simulink model "FILTRE_KALMAN_Design"  (R2024a)
settings: Solver=FixedStepAuto  StartTime=0.0  StopTime=10.0  FixedStep=0.01  RelTol=1e-3
values from neighbouring files (symbols this model uses):
  A = [0 0 1 0; 0 0 0 1; 0 aa -bb -cc; 0 dd -ee -ff]    [Init_Setup.m]
  b = 0.00007892    (= 7.892e-05)    [Init_Setup.m]
  B = [0;0; mm; nn]    [Init_Setup.m]
  c = 0.63    [Init_Setup.m]
  C = eye(4)    [Init_Setup.m]
  D = [0 0 0 0]'    [Init_Setup.m]
  g = 9.81    [Init_Setup.m]
  I = 0.0007176    [Init_Setup.m]
  kb = 0.031    [Init_Setup.m]
  kt = 0.031    [Init_Setup.m]
  l = 0.2    [Init_Setup.m]
  M = 0.136    [Init_Setup.m]
  m = 0.1    [Init_Setup.m]
  r = 0.006    [Init_Setup.m]
  Rm = 12.5    [Init_Setup.m]
undefined symbols (not defined in the file or in its folder): Continuous, Time
libraries: simulink x2, ctrlSharedLib x1
settings Model: Creator=jitendra  LastModifiedBy=USER
settings SolverCC: AlgebraicLoopSolver=TrustRegion
settings DataIOCC: ExternalInput=getinputstruct(op_trim1)  InitialState=getstatestruct(op_trim1)  ReturnWorkspaceOutputs=off
settings DebuggingCC: UnconnectedInputMsg=warning  UnconnectedOutputMsg=warning  UnconnectedLineMsg=warning  ArithmeticOperatorsInVariantConditions=warning
settings ModelReferenceCC: EnableRefExpFcnMdlSchedulingChecks=on
settings SFSimCC: SimUseLocalCustomCode=off  CustomCodeUndefinedFunction=UseInterfaceOnly
settings RTWCC: RTWUseLocalCustomCode=off  GPUComputeCapability=3.5

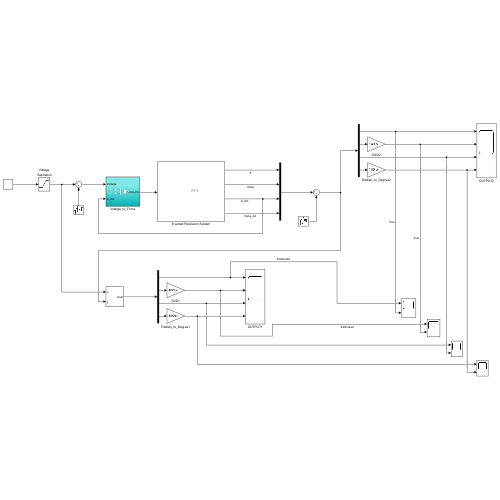
[thumbnail: Simulink's stored preview of the top-level diagram]
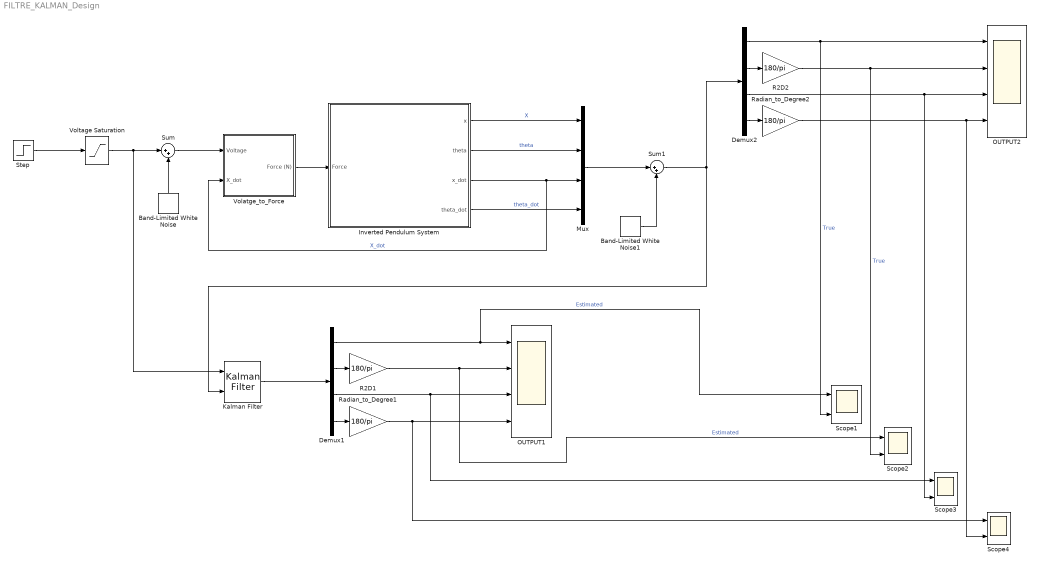
== system FILTRE_KALMAN_Design ==
  Band-Limited White Noise : simulink/Sources/Band-Limited White Noise  Cov=[0.000015]  Ts=0.1  seed=[23341]
  Band-Limited White Noise1 : simulink/Sources/Band-Limited White Noise  Cov=[0.00015]  Ts=0.1  seed=[23341]
  Demux1 : Demux
  Demux2 : Demux
  Inverted Pendulum System : Subsystem
      mask Display: image('ip_model.png');
  Kalman Filter : ctrlSharedLib/Kalman Filter  TimeDomain=Continuous-Time  UseCurrentEstimator=on  ModelSource=Individual A, B, C, D matrices  ModelSourceVariable=ss(0.95,1,1,0,1)  A=A  B=B  C=C  D=D  NumberOfStates=1  NumberOfInputs=1  NumberOfOutputs=1  InitialEstimateSource=Dialog  X0=0  P0=10  UseK=off  UseGH=off  NumberOfProcessNoiseInputs=1  G=1  TimeInvariantG=on  H=0  TimeInvariantH=on  Q=0.05  TimeInvariantQ=on  R=1  TimeInvariantR=on  N=0  TimeInvariantN=on  AddInputPort=on  AddEnablePort=off  OutputEstimatedY=off  OutputP=off  Ts=-1
  Mux : Mux
  OUTPUT1 : Scope  NumInputPorts=4
  OUTPUT2 : Scope  NumInputPorts=4
  R2D1 : Gain  Gain=180/pi
  R2D2 : Gain  Gain=180/pi
  Radian_to_Degree1 : Gain  Gain=180/pi
  Radian_to_Degree2 : Gain  Gain=180/pi
  Scope{1..4} (4 alike) : Scope  NumInputPorts=2
  Step : Step  SampleTime=0
  Sum : Sum  Inputs=|++
  Sum1 : Sum  Inputs=|++
  Volatge_to_Force : Subsystem
  Voltage Saturation : Saturate  UpperLimit=12  LowerLimit=-12
  wires:
  Inverted Pendulum System/3(x_dot) -> Volatge_to_Force/2(X_dot), Mux/3  "X_dot"
  Inverted Pendulum System/2(theta) -> Mux/2  "theta"
  Inverted Pendulum System/1(x) -> Mux/1  "X"
  Inverted Pendulum System/4(theta_dot) -> Mux/4  "theta_dot"
  Mux/1 -> Sum1/1
  Volatge_to_Force/1(Force (N)) -> Inverted Pendulum System/1(Force)
  Step/1 -> Voltage Saturation/1
  Sum/1 -> Volatge_to_Force/1(Voltage)
  Band-Limited White Noise/1 -> Sum/2
  Voltage Saturation/1 -> Sum/1, Kalman Filter/1
  Band-Limited White Noise1/1 -> Sum1/2
  Radian_to_Degree1/1 -> Scope4/1, OUTPUT1/4
  Demux1/4 -> Radian_to_Degree1/1
  R2D1/1 -> Scope2/1, OUTPUT1/2  "Estimated"
  Demux1/2 -> R2D1/1
  Demux1/1 -> Scope1/1, OUTPUT1/1  "Estimated"
  Demux1/3 -> OUTPUT1/3, Scope3/1
  Kalman Filter/1 -> Demux1/1
  Demux2/4 -> Radian_to_Degree2/1
  Sum1/1 -> Kalman Filter/2, Demux2/1
  Demux2/2 -> R2D2/1
  R2D2/1 -> Scope2/2, OUTPUT2/2  "True"
  Demux2/1 -> OUTPUT2/1, Scope1/2  "True"
  Demux2/3 -> Scope3/2, OUTPUT2/3
  Radian_to_Degree2/1 -> Scope4/2, OUTPUT2/4

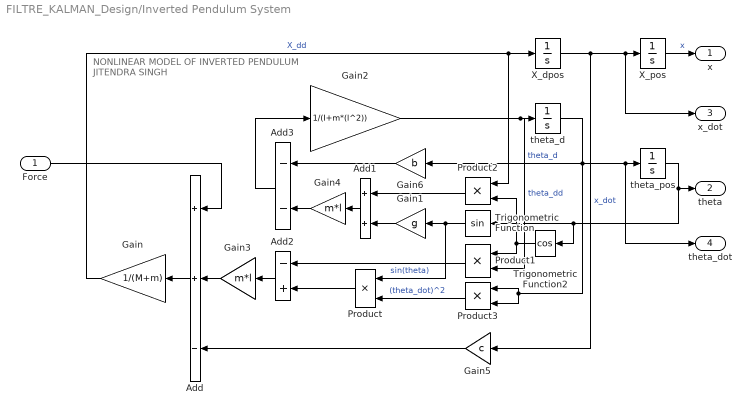
== system FILTRE_KALMAN_Design/Inverted Pendulum System ==
  note: NONLINEAR MODEL OF
      | INVERTED PENDULUM
      | JITENDRA SINGH
  Force : Inport
  Add : Sum  Inputs=++-
  Add1 : Sum
  Add2 : Sum  Inputs=-+
  Add3 : Sum  Inputs=--
  Gain : Gain  Gain=1/(M+m)
  Gain1 : Gain  Gain=g
  Gain2 : Gain  Gain=1/(I+m*(l^2))
  Gain3 : Gain  Gain=m*l
  Gain4 : Gain  Gain=m*l
  Gain5 : Gain  Gain=c
  Gain6 : Gain  Gain=b
  Product{,1..3} (4 alike) : Product
  Trigonometric Function : Trigonometry
  Trigonometric Function2 : Trigonometry  Operator=cos
  X_dpos : Integrator
  X_pos : Integrator  InitialCondition=0.2
  theta_d : Integrator
  theta_pos : Integrator  InitialCondition=160*(pi/180)
  x : Outport  VectorParamsAs1DForOutWhenUnconnected=off
  theta : Outport  Port=2  VectorParamsAs1DForOutWhenUnconnected=off
  x_dot : Outport  Port=3  VectorParamsAs1DForOutWhenUnconnected=off
  theta_dot : Outport  Port=4  VectorParamsAs1DForOutWhenUnconnected=off
  wires:
  Gain5/1 -> Add/3
  Add2/1 -> Gain3/1
  Add3/1 -> Gain2/1
  Trigonometric Function2/1 -> Product2/2, Product1/1
  Trigonometric Function/1 -> Product/1, Gain1/1  "sin(theta)"
  Gain3/1 -> Add/2
  theta_d/1 -> Product3/2, Product3/1, Gain6/1, theta_dot/1, theta_pos/1  "theta_d"
  Product2/1 -> Add1/1
  Product/1 -> Add2/2
  Gain4/1 -> Add3/2
  Product3/1 -> Product/2  "(theta_dot)^2"
  X_pos/1 -> x/1  "x"
  Product1/1 -> Add2/1
  Gain/1 -> X_dpos/1, Product2/1  "X_dd"
  Add/1 -> Gain/1
  Gain2/1 -> Product1/2, theta_d/1  "theta_dd"
  Gain6/1 -> Add3/1
  theta_pos/1 -> Trigonometric Function2/1, Trigonometric Function/1, theta/1
  Force/1 -> Add/1
  Gain1/1 -> Add1/2
  X_dpos/1 -> x_dot/1, X_pos/1, Gain5/1  "x_dot"
  Add1/1 -> Gain4/1

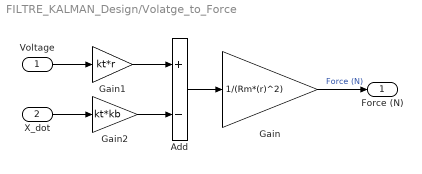
== system FILTRE_KALMAN_Design/Volatge_to_Force ==
  Voltage : Inport
  X_dot : Inport  Port=2
  Add : Sum  Inputs=+-
  Gain : Gain  Gain=1/(Rm*(r)^2)
  Gain1 : Gain  Gain=kt*r
  Gain2 : Gain  Gain=kt*kb
  Force (N) : Outport  VectorParamsAs1DForOutWhenUnconnected=off
  wires:
  Gain1/1 -> Add/1
  Gain2/1 -> Add/2
  Voltage/1 -> Gain1/1
  Gain/1 -> Force (N)/1  "Force (N)"
  X_dot/1 -> Gain2/1
  Add/1 -> Gain/1
